simulink model "cte_elect"  (Simulink 6.1)
settings: Solver=ode23tb  SolverMode=SingleTasking  StartTime=0  StopTime=200e-3  MaxStep=1e-6
libraries: powerlib2 x9
settings Model: LastModifiedBy=Administrador  ExtModeTrigMode=oneshot  ExtModeArmWhenConnect=off
settings DataIOCC: LimitDataPoints=off  SaveFinalState=on  SaveOutput=off  SaveTime=off  SignalLoggingName=sigsOut
settings OptimizationCC: BlockReduction=off  BooleanDataType=off
settings DebuggingCC: UnconnectedInputMsg=none  UnconnectedOutputMsg=none
settings HardwareCC: TargetUnknown=on
settings RTWCC: TemplateMakefile=grt_unix.tmf

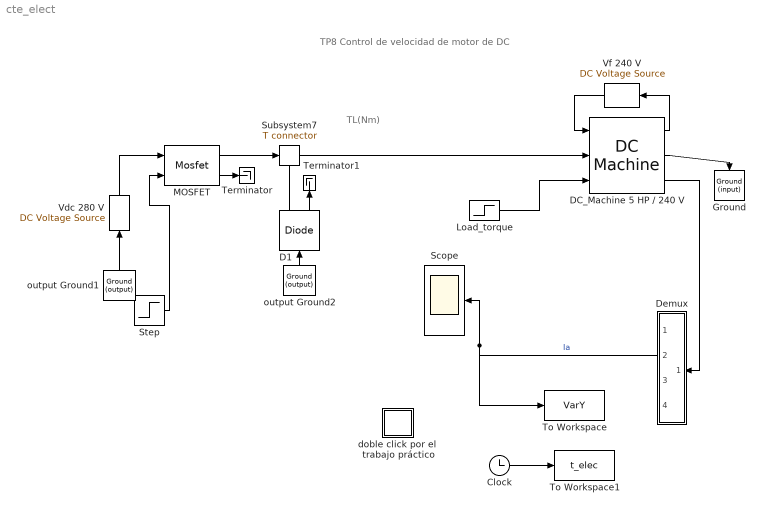
== system cte_elect ==
  note: TL(Nm)
  note: TP8 Control de velocidad de motor de DC
  Clock : Clock
      settings: Decimation=10
  D1 : powerlib2/Power Electronics/Diode  Tag=PoWeRsYsTeMbLoCk  Orientation=up  Ron=0.05  Lon=5e-6  Vf=0.7  IC=0  Rs=Inf  Cs=0.1e-6  PSBOutputType=10
  DC_Machine 5 HP / 240 V : powerlib2/Machines/DC Machine  RLa="[0.5  0.01]"  RLf="[240  0]"  Laf=1.23  J=0.05  Bm=2000  Tf=0  w0=1e-1  PSBOutputType=110
  Demux : Subsystem  Orientation=left
  Ground : powerlib2/Connectors/Ground (input)  Tag=PoWeRsYsTeMbLoCk  Orientation=down
  "Load_torque " : Step  Time=0  After=0  SampleTime=0
  MOSFET : powerlib2/Power Electronics/Mosfet  Tag=PoWeRsYsTeMbLoCk  Ron=0.001  Lon=1e-6  Rd=.001  IC=0  Rs=10  Cs=0.01e-6  PSBOutputType=10
  Scope : Scope
      settings: TickLabels=on  TimeRange=0.2  YMin=0  YMax=600  SaveName=var  Decimation=20
  Step : Step  Time=0.000001  After=3  SampleTime=0
  Subsystem7 : powerlib2/Connectors/T connector  Tag=PoWeRsYsTeMbLoCk  PSBOutputType=1
  Terminator : Terminator
  Terminator1 : Terminator
      settings: Orientation=up
  To Workspace : ToWorkspace  VariableName=VarY  SampleTime=-1  SaveFormat=Array
  To Workspace1 : ToWorkspace  VariableName=t_elec  SampleTime=-1  SaveFormat=Array
  "Vdc 280 V " : powerlib2/Electrical Sources/DC Voltage Source  Tag=PoWeRsYsTeMbLoCk  Orientation=up  V=280  mesure=None  PSBOutputType=1
  Vf 240 V : powerlib2/Electrical Sources/DC Voltage Source  Tag=PoWeRsYsTeMbLoCk  Orientation=left  V=240  mesure=None  PSBOutputType=1
  doble click por el  trabajo práctico : Subsystem
      mask Display: disp('?')
  output Ground1 : powerlib2/Connectors/Ground (output)  Tag=PoWeRsYsTeMbLoCk  Orientation=up  PSBOutputType=1
  output Ground2 : powerlib2/Connectors/Ground (output)  Tag=PoWeRsYsTeMbLoCk  Orientation=up  PSBOutputType=1
  wires:
  D1/2 -> Terminator1/1
  MOSFET/2 -> Terminator/1
  output Ground2/1 -> D1/1
  D1/1 -> Subsystem7/Enable
  MOSFET/1 -> Subsystem7/1
  "Vdc 280 V "/1 -> MOSFET/1
  output Ground1/1 -> "Vdc 280 V "/1
  Vf 240 V/1 -> DC_Machine 5 HP / 240 V/1
  DC_Machine 5 HP / 240 V/2 -> Ground/1
  DC_Machine 5 HP / 240 V/1 -> Vf 240 V/1
  DC_Machine 5 HP / 240 V/3 -> Demux/1(m)
  Step/1 -> MOSFET/2
  "Load_torque "/1 -> DC_Machine 5 HP / 240 V/3
  Subsystem7/1 -> DC_Machine 5 HP / 240 V/2
  Demux/2(Ia) -> Scope/1, To Workspace/1  "Ia"
  Clock/1 -> To Workspace1/1

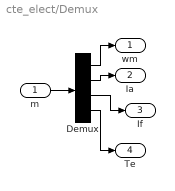
== system cte_elect/Demux ==
  m : Inport  Port=1  LatchInput=off
  Demux : Demux
  wm : Outport
  Ia : Outport  Port=2
  If : Outport  Port=3
  Te : Outport  Port=4
  wires:
  Demux/1 -> wm/1
  Demux/2 -> Ia/1
  m/1 -> Demux/1
  Demux/3 -> If/1
  Demux/4 -> Te/1

== system cte_elect/doble click por el  trabajo práctico ==
  note: Ejecute la simulación. Observe en el osciloscopio la tensión del motor, corriente, velocidad y par.
      |
      | La referencia de velocidad es un escalón que comienza con wm = 120 rad/s y en el instante de tiempo (0,4s)
      | cambia por wm = 120 rad/s.
      |
      | El par cambia con forma de escalón desde el valor inicial TL = 5 N.m a Te = 25 N.m en 1,2 seg.
  note: TP 8; Case study I: Chopper-Fed DC Motor Drive
  note: Circuit description
  note: Womework
  note: El motor de DC está alimentado por un chopper de DC con MOSFET operando en clase A.
      | La carga mecánica está caracterizada por un escalón de carga TL.
      |
      | El controlador de corriente de histéresis compara la corriente sensada con una referencia y genera la señal de compuerta
      | del MOSFET forzando al motor a seguir la corriente de referencia.
      | El lazo de velocidad utiliza un controlador PI que produce la referencia para el lazo de corriente (par).
      | El bloque de Voltage Measurement provee señal para los propositos de visualización.
  note: (Modificado del archivo original de H. Le-Huy, Université Laval, Québec)
  note: Measurements
  note: a) Imprima las magnitudes medidas en osciloscopio
      | b) Mida la constante de tiempo eléctrica del motor
      | c) Mida la constante de tiempo mecánica del motor
      | d) Cambie los valores del controlador (speed controller)
      | y busque (prueba y error) la sintonización más óptima,
      | sin cambiar el límite de corriente.
  note: Conclusion
  note: a) acerca de las constantes de tiempo
      | b) acerca de la ecuación general de par Te=TL+J*d(wm)/dt
      | c) Acerca del controlador (speed controller)
      | d) generales (otros)
